simulink model "murad_nmpc"  (R2019a)
settings: Solver=FixedStepAuto  StartTime=0.0  StopTime=440  FixedStep=.001  MaxStep=0.01  RelTol=1e-3
libraries: simulink_extras x2, Solver_SF x1
settings Model: SimulationMode=accelerator  Creator=Murad  LastModifiedBy=Murad
settings SolverCC: AlgebraicLoopSolver=LineSearch
settings OptimizationCC: EfficientMapNaN2IntZero=off
settings HardwareCC: TargetBitPerPointer=64  TargetBitPerSizeT=64  TargetBitPerPtrDiffT=64  TargetLongLongMode=on  TargetIntDivRoundTo=Zero  TargetEndianess=LittleEndian  TargetWordSize=64  TargetHWDeviceType=MATLAB Host  ProdEqTarget=off
settings CodeAppCC: MaxIdLength=128
settings GRTTargetCC: TargetLangStandard=C89/C90 (ANSI)  GRTInterface=on

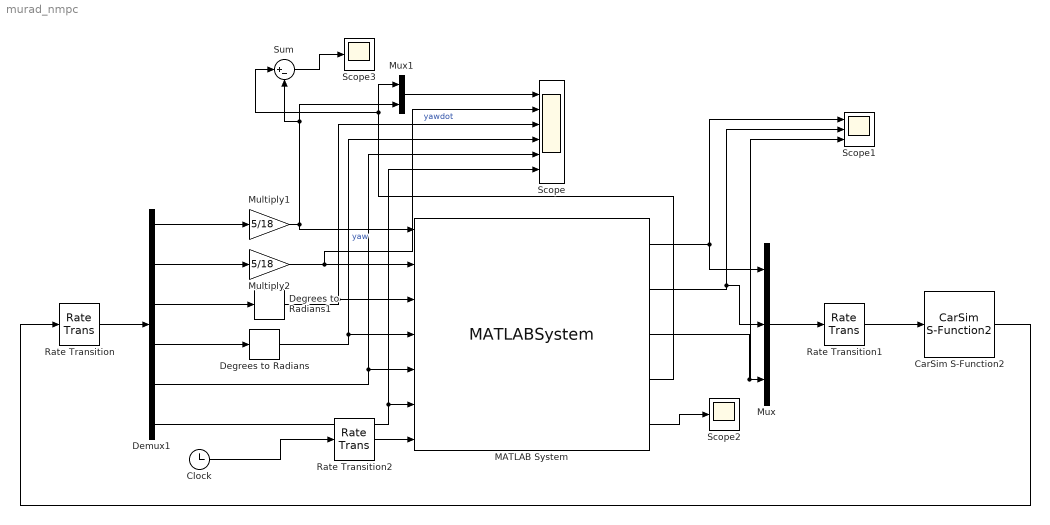
== system murad_nmpc ==
  CarSim S-Function2 : Solver_SF/CarSim S-Function2  Priority=1  VehicleCode=i_s  SIMFILE=nmpc.sim
      settings: AttributesFormatString=Vehicle Code: %<VehicleCode>
  Clock : Clock
  Degrees to Radians : simulink_extras/Transformations/Degrees to Radians
  Degrees to Radians1 : simulink_extras/Transformations/Degrees to Radians
  Demux1 : Demux  Outputs=6
  MATLAB System : MATLABSystem  System=casadi_block_presented  SimulateUsing=Interpreted execution
      mask Type: casadi_block_presented
      mask Display:
      | disp('casadi_block_presented');
      | port_label('input',1,'xd_in');
      | port_label('input',2,'yd_in');
      | port_label('input',3,'yawd_in');
      | port_label('input',4,'yaw_in');
      | port_label('input',5,'x_in');
      | port_label('input',6,'y_in');
      | port_label('input',7,'t');
      | port_label('output',1,'delta_out');
      | port_label('output',2,'acc_out');
      | port_label('output',3,'break_out');
      | port_label('output',4,'vref');
      | port_label('output',5,'err');
  Multiply1 : Gain  Gain=5/18
  Multiply2 : Gain  Gain=5/18
  Mux : Mux  Inputs=3
  Mux1 : Mux  Inputs=2
  Rate Transition : RateTransition  OutPortSampleTime=0.02
  Rate Transition1 : RateTransition  OutPortSampleTime=0.001
  Rate Transition2 : RateTransition  OutPortSampleTime=0.02
  Scope : Scope  NumInputPorts=6
  Scope1 : Scope  NumInputPorts=3
  Scope2 : Scope
  Scope3 : Scope
  Sum : Sum  Inputs=|+-
  wires:
  Multiply1/1 -> Sum/2, Mux1/2, MATLAB System/1
  MATLAB System/3 -> Scope1/3, Mux/3
  Degrees to Radians/1 -> Scope/4, MATLAB System/4  "yaw"
  Demux1/3 -> Degrees to Radians1/1
  Demux1/2 -> Multiply2/1
  MATLAB System/1 -> Mux/1, Scope1/1
  Demux1/1 -> Multiply1/1
  Degrees to Radians1/1 -> Scope/3, MATLAB System/3  "yawdot"
  Multiply2/1 -> Scope/2, MATLAB System/2
  Demux1/4 -> Degrees to Radians/1
  Demux1/5 -> Scope/5, MATLAB System/5
  CarSim S-Function2/1 -> Rate Transition/1
  Demux1/6 -> Scope/6, MATLAB System/6
  Mux/1 -> Rate Transition1/1
  Clock/1 -> Rate Transition2/1
  Mux1/1 -> Scope/1
  MATLAB System/5 -> Scope2/1
  MATLAB System/2 -> Mux/2, Scope1/2
  MATLAB System/4 -> Sum/1, Mux1/1
  Sum/1 -> Scope3/1
  Rate Transition/1 -> Demux1/1
  Rate Transition1/1 -> CarSim S-Function2/1
  Rate Transition2/1 -> MATLAB System/7
